simulink model "myelosuppression_model"  (R2020a)
settings: Solver=VariableStepAuto  StartTime=0.0  StopTime=50.0  RelTol=1e-3
values from neighbouring files (symbols this model uses):
  circ0 = 5.04    [project3.m]
  Edrugss = Edrugf    (= 0.176268421044)    [project3.m]
  gamma = 0.16    [project3.m]
  kcirc = 4/120.4    (= 0.0332225913621)    [project3.m]
  ktr = 4/120.4    (= 0.0332225913621)    [project3.m]
settings Model: Creator=Alan  LastModifiedBy=Alan

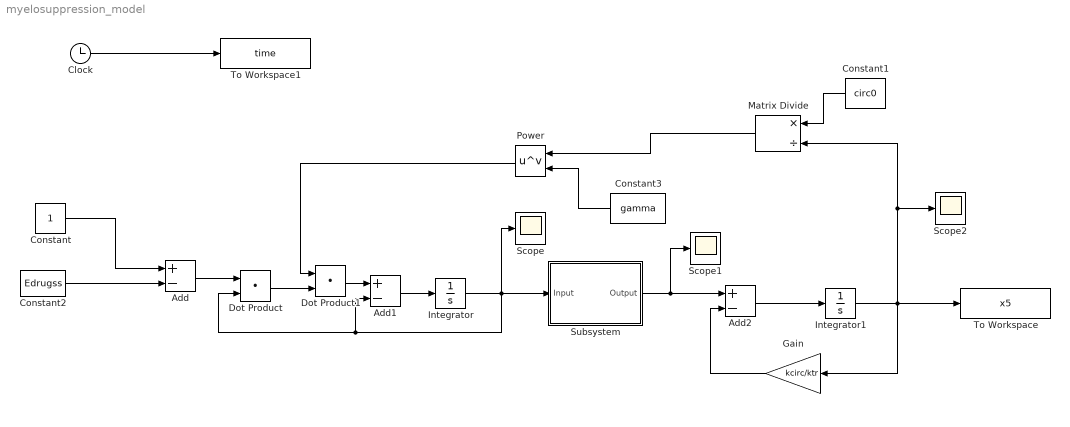
== system myelosuppression_model ==
  Add : Sum  Inputs=+-
  Add1 : Sum  Inputs=+-
  Add2 : Sum  Inputs=+-
  Clock : Clock
  Constant : Constant
  Constant1 : Constant  Value=circ0
  Constant2 : Constant  Value=Edrugss
  Constant3 : Constant  Value=gamma
  Dot Product : DotProduct  OutDataTypeStr=Inherit: Inherit via internal rule
  Dot Product1 : DotProduct  OutDataTypeStr=Inherit: Inherit via internal rule
  Gain : Gain  Gain=kcirc/ktr
  Integrator : Integrator  InitialCondition=circ0
  Integrator1 : Integrator  InitialCondition=circ0
  Matrix Divide : Product  Inputs=*/
  Power : Math  Operator=pow  SaturateOnIntegerOverflow=on
  Scope : Scope
  Scope1 : Scope
  Scope2 : Scope
  Subsystem : Subsystem
  To Workspace : ToWorkspace  VariableName=x5  SaveFormat=Timeseries  SampleTime=-1
  To Workspace1 : ToWorkspace  VariableName=time  SaveFormat=Timeseries  SampleTime=-1
  wires:
  Constant2/1 -> Add/2
  Constant/1 -> Add/1
  Add/1 -> Dot Product/1
  Dot Product/1 -> Dot Product1/2
  Power/1 -> Dot Product1/1
  Constant3/1 -> Power/2
  Dot Product1/1 -> Add1/1
  Add1/1 -> Integrator/1
  Integrator/1 -> Scope/1, Dot Product/2, Add1/2, Subsystem/1(Input)
  Constant1/1 -> Matrix Divide/1
  Matrix Divide/1 -> Power/1
  Subsystem/1(Output) -> Scope1/1, Add2/1
  Gain/1 -> Add2/2
  Add2/1 -> Integrator1/1
  Integrator1/1 -> Matrix Divide/2, Scope2/1, Gain/1, To Workspace/1
  Clock/1 -> To Workspace1/1

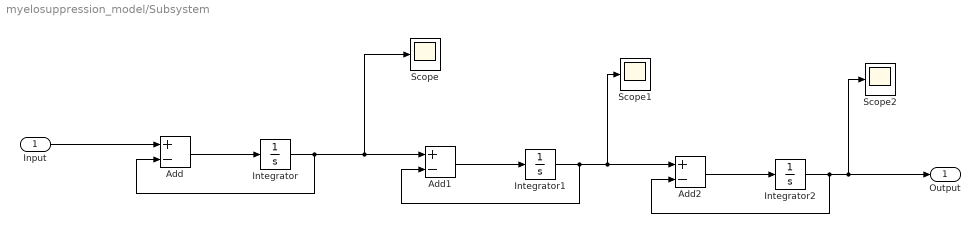
== system myelosuppression_model/Subsystem ==
  Input : Inport
  Add : Sum  Inputs=+-
  Add1 : Sum  Inputs=+-
  Add2 : Sum  Inputs=+-
  Integrator : Integrator  InitialCondition=circ0
  Integrator1 : Integrator  InitialCondition=circ0
  Integrator2 : Integrator  InitialCondition=circ0
  Scope : Scope
  Scope1 : Scope
  Scope2 : Scope
  Output : Outport
  wires:
  Add2/1 -> Integrator2/1
  Integrator1/1 -> Scope1/1, Add2/1, Add1/2
  Integrator/1 -> Add/2, Scope/1, Add1/1
  Add1/1 -> Integrator1/1
  Input/1 -> Add/1
  Add/1 -> Integrator/1
  Integrator2/1 -> Scope2/1, Output/1, Add2/2
